simulink library "INT_Rail_CtlLoop"  (R2016b)
settings: Solver=VariableStepAuto  StartTime=0.0  StopTime=10.0  RelTol=1e-3
settings Model: Creator=liutao  LastModifiedBy=liutao

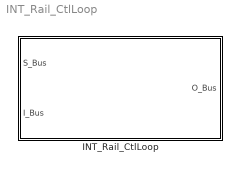
== system INT_Rail_CtlLoop ==
  INT_Rail_CtlLoop : Subsystem

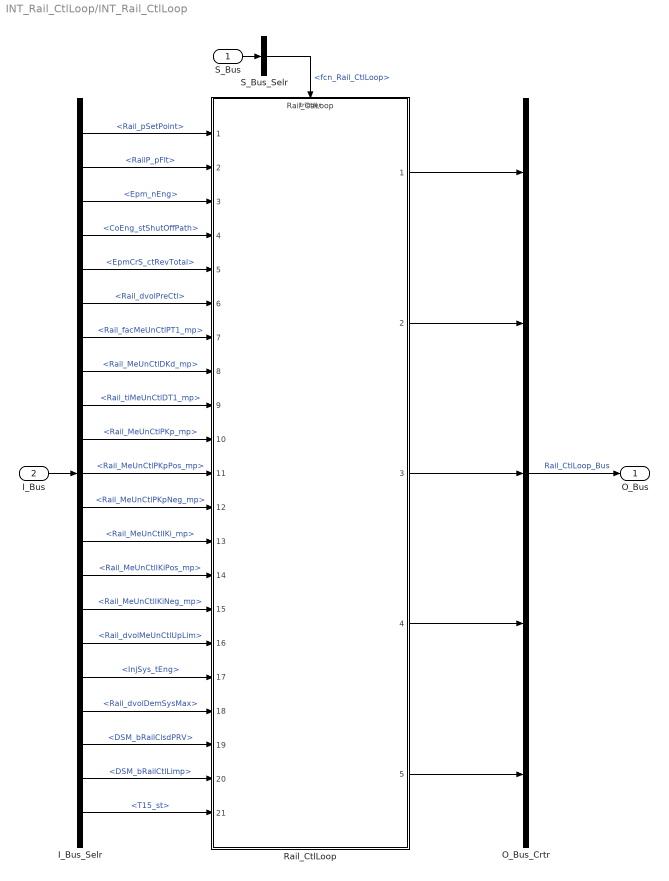
== system INT_Rail_CtlLoop/INT_Rail_CtlLoop ==
  S_Bus : Inport
  I_Bus : Inport  Port=2
  I_Bus_Selr : BusSelector  OutputSignals=Rail_pSetPoint,RailP_pFlt,Epm_nEng,CoEng_stShutOffPath,EpmCrS_ctRevTotal,Rail_dvolPreCtl,Rail_facMeUnCtlPT1_mp,Rail_MeUnCtlDKd_mp,Rail_tiMeUnCtlDT1_mp,Rail_MeUnCtlPKp_mp,Rail_MeUnCtlPKpPos_mp,Rail_MeUnCtlPKpNeg_mp,Rail_MeUnCtlIKi_mp,Rail_MeUnCtlIKiPos_mp,Rail_MeUnCtlIKiNeg_mp,Rail_dvolMeUnCtlUpLim,InjSys_tEng,Rail_dvolDemSysMax,DSM_bRailClsdPRV,DSM_bRailCtlLimp,T15_st
  O_Bus_Crtr : BusCreator  Inputs=5
  Rail_CtlLoop : ModelReference  ModelNameDialog=Rail_CtlLoop  SimulationMode=Normal  ModelReferenceVersion=1.34  TriggerPortName=function  TriggerPortTriggerType=function-call  TriggerPortStatesWhenEnabling=held
  S_Bus_Selr : BusSelector  OutputSignals=fcn_Rail_CtlLoop
  O_Bus : Outport
  wires:
  S_Bus_Selr/1 -> Rail_CtlLoop/Trigger  "<fcn_Rail_CtlLoop>"
  S_Bus/1 -> S_Bus_Selr/1
  I_Bus/1 -> I_Bus_Selr/1
  I_Bus_Selr/1 -> Rail_CtlLoop/1  "<Rail_pSetPoint>"
  I_Bus_Selr/2 -> Rail_CtlLoop/2  "<RailP_pFlt>"
  I_Bus_Selr/3 -> Rail_CtlLoop/3  "<Epm_nEng>"
  I_Bus_Selr/4 -> Rail_CtlLoop/4  "<CoEng_stShutOffPath>"
  I_Bus_Selr/5 -> Rail_CtlLoop/5  "<EpmCrS_ctRevTotal>"
  I_Bus_Selr/6 -> Rail_CtlLoop/6  "<Rail_dvolPreCtl>"
  I_Bus_Selr/7 -> Rail_CtlLoop/7  "<Rail_facMeUnCtlPT1_mp>"
  I_Bus_Selr/8 -> Rail_CtlLoop/8  "<Rail_MeUnCtlDKd_mp>"
  I_Bus_Selr/9 -> Rail_CtlLoop/9  "<Rail_tiMeUnCtlDT1_mp>"
  I_Bus_Selr/10 -> Rail_CtlLoop/10  "<Rail_MeUnCtlPKp_mp>"
  I_Bus_Selr/11 -> Rail_CtlLoop/11  "<Rail_MeUnCtlPKpPos_mp>"
  I_Bus_Selr/12 -> Rail_CtlLoop/12  "<Rail_MeUnCtlPKpNeg_mp>"
  I_Bus_Selr/13 -> Rail_CtlLoop/13  "<Rail_MeUnCtlIKi_mp>"
  I_Bus_Selr/14 -> Rail_CtlLoop/14  "<Rail_MeUnCtlIKiPos_mp>"
  I_Bus_Selr/15 -> Rail_CtlLoop/15  "<Rail_MeUnCtlIKiNeg_mp>"
  I_Bus_Selr/16 -> Rail_CtlLoop/16  "<Rail_dvolMeUnCtlUpLim>"
  I_Bus_Selr/17 -> Rail_CtlLoop/17  "<InjSys_tEng>"
  I_Bus_Selr/18 -> Rail_CtlLoop/18  "<Rail_dvolDemSysMax>"
  I_Bus_Selr/19 -> Rail_CtlLoop/19  "<DSM_bRailClsdPRV>"
  I_Bus_Selr/20 -> Rail_CtlLoop/20  "<DSM_bRailCtlLimp>"
  I_Bus_Selr/21 -> Rail_CtlLoop/21  "<T15_st>"
  O_Bus_Crtr/1 -> O_Bus/1  "Rail_CtlLoop_Bus"
  Rail_CtlLoop/1 -> O_Bus_Crtr/1
  Rail_CtlLoop/2 -> O_Bus_Crtr/2
  Rail_CtlLoop/3 -> O_Bus_Crtr/3
  Rail_CtlLoop/4 -> O_Bus_Crtr/4
  Rail_CtlLoop/5 -> O_Bus_Crtr/5
